simulink model "lab7_2_sym"  (R2021a)
settings: Solver=ode45  StartTime=0.0  StopTime=15.0  MaxStep=2^(-5)  RelTol=1e-3
settings Model: Creator=sheil  LastModifiedBy=sheil

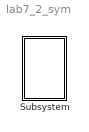
== system lab7_2_sym ==
  Subsystem : Subsystem  mask{g=9.81, k1=2, k2=1, m1=1, m2=2, l1=1, l2=2, t10=80, t20=150, t11=0, t21=0}
      mask prompts: g "przyspieszenie"; k1 "wsp. tlumienia 1"; k2 "wsp. tlumienia 2"; m1 "masa wahadla 1"; m2 "masa wahadla 2"; l1 "dlugosc linki 1"; l2 "dlugosc linki 2"; t10 "kat wychylenia wahadla 1"; t20 "kat wychylenia wahadla 2"; t11 "predkosc wahadla"; t21 "predkosc wahadla 2"

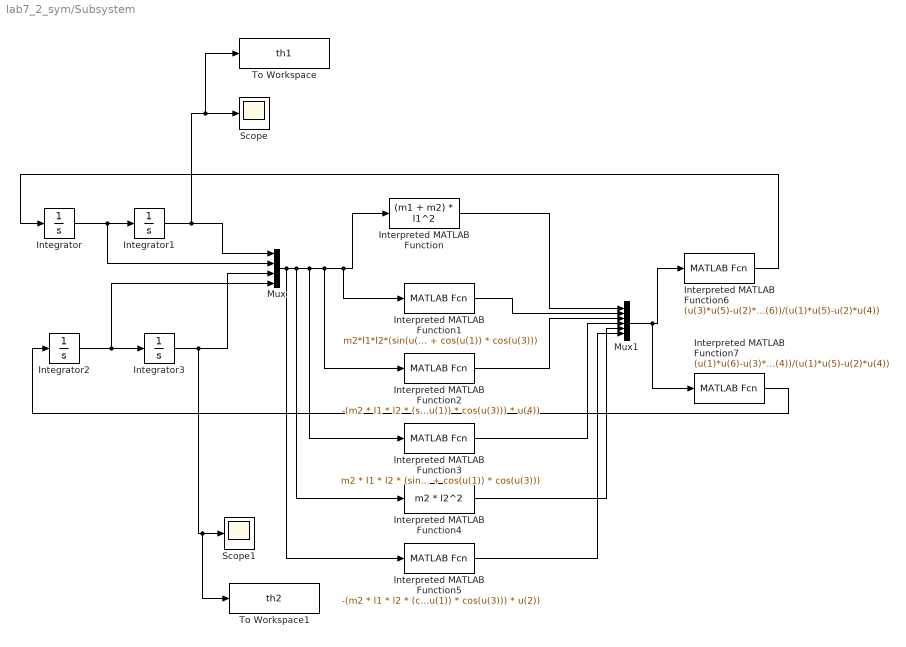
== system lab7_2_sym/Subsystem ==
  Integrator : Integrator  InitialCondition=t11*pi/180
  Integrator1 : Integrator  InitialCondition=t10*pi/180
  Integrator2 : Integrator  InitialCondition=t21*pi/180
  Integrator3 : Integrator  InitialCondition=t20*pi/180
  Interpreted MATLAB Function : MATLABFcn  MATLABFcn=(m1 + m2) * l1^2  OutputDimensions=1
  Interpreted MATLAB Function1 : MATLABFcn  MATLABFcn=m2*l1*l2*(sin(u(1)) * sin(u(3)) + cos(u(1)) * cos(u(3)))  OutputDimensions=1
  Interpreted MATLAB Function2 : MATLABFcn  MATLABFcn=-(m2 * l1 * l2 * (sin(u(1)) * cos(u(3)) - cos(u(1)) * sin(u(3))) * u(4)^2 + (m1 + m2) * g * l1 * sin(u(1)) + k1 * l1^2 * u(2) + k2 * l1 * l2 * (sin(u(1)) * sin(u(3)) + cos(u(1)) * cos(u(3))) * u(4))  OutputDimensions=1
  Interpreted MATLAB Function3 : MATLABFcn  MATLABFcn=m2 * l1 * l2 * (sin(u(1)) * sin(u(3)) + cos(u(1)) * cos(u(3)))  OutputDimensions=1
  Interpreted MATLAB Function4 : MATLABFcn  MATLABFcn=m2 * l2^2  OutputDimensions=1
  Interpreted MATLAB Function5 : MATLABFcn  MATLABFcn=-(m2 * l1 * l2 * (cos(u(1)) * sin(u(3)) - sin(u(1)) * cos(u(3))) * u(2)^2 + m2 * g * l2 * sin(u(3)) + k2 * l2^2 * u(4) + k2 * l1 * l2 *(sin(u(1)) * sin(u(3)) + cos(u(1)) * cos(u(3))) * u(2))  OutputDimensions=1
  Interpreted MATLAB Function6 : MATLABFcn  MATLABFcn=(u(3)*u(5)-u(2)*u(6))/(u(1)*u(5)-u(2)*u(4))  OutputDimensions=1
  Interpreted MATLAB Function7 : MATLABFcn  MATLABFcn=(u(1)*u(6)-u(3)*u(4))/(u(1)*u(5)-u(2)*u(4))  OutputDimensions=1
  Mux : Mux
  Mux1 : Mux  Inputs=6
  Scope : Scope
  Scope1 : Scope
  To Workspace : ToWorkspace  VariableName=th1  SampleTime=-1
  To Workspace1 : ToWorkspace  VariableName=th2  SampleTime=-1
  wires:
  Interpreted MATLAB Function5/1 -> Mux1/6
  Interpreted MATLAB Function2/1 -> Mux1/3
  Integrator/1 -> Mux/2, Integrator1/1
  Integrator2/1 -> Mux/4, Integrator3/1
  Interpreted MATLAB Function4/1 -> Mux1/5
  Mux1/1 -> Interpreted MATLAB Function7/1, Interpreted MATLAB Function6/1
  Mux/1 -> Interpreted MATLAB Function5/1, Interpreted MATLAB Function4/1, Interpreted MATLAB Function3/1, Interpreted MATLAB Function2/1, Interpreted MATLAB Function1/1, Interpreted MATLAB Function/1
  Interpreted MATLAB Function6/1 -> Integrator/1
  Interpreted MATLAB Function3/1 -> Mux1/4
  Interpreted MATLAB Function7/1 -> Integrator2/1
  Interpreted MATLAB Function1/1 -> Mux1/2
  Integrator3/1 -> To Workspace1/1, Scope1/1, Mux/3
  Integrator1/1 -> To Workspace/1, Scope/1, Mux/1
  Interpreted MATLAB Function/1 -> Mux1/1
